simulink model "SimulinkSS"  (R2019a)
settings: Solver=FixedStepAuto  StartTime=0.0  StopTime=60  FixedStep=1e-2  RelTol=1e-3
undefined symbols (not defined in the file): G, K, Ki, x0_tf4
settings Model: Creator=luisg  LastModifiedBy=luisg

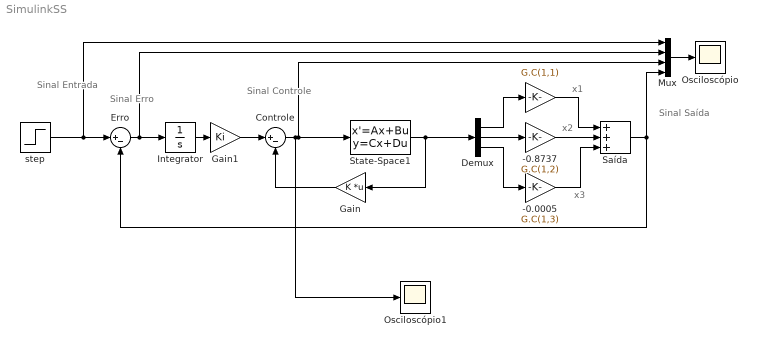
== system SimulinkSS ==
  note: Sinal
      | Entrada
  note: x1
  note: x2
  note: x3
  note: Sinal
      | Erro
  note: Sinal
      | Controle
  note: Sinal
      | Saída
  " " : Gain  Gain=G.C(1,1)
  -0.0005 : Gain  Gain=G.C(1,3)
  -0.8737 : Gain  Gain=G.C(1,2)
  Controle : Sum  Inputs=|+-
  Demux : Demux  Outputs=3
  Erro : Sum  Inputs=|+-
  Gain : Gain  Gain=K  Multiplication=Matrix(K*u)
  Gain1 : Gain  Gain=Ki
  Integrator : Integrator
  Mux : Mux
  Osciloscópio : Scope
  Osciloscópio1 : Scope
  Saída : Sum  Inputs=+++
  State-Space1 : StateSpace  A=G.A  B=G.B  C=[1 0 0; 0 1 0; 0 0 1]  D=[0;0;0]  InitialCondition=x0_tf4
  step : Step  Time=100  Before=70  After=70  SampleTime=0.05
  wires:
  Controle/1 -> State-Space1/1, Mux/3, Osciloscópio1/1
  Gain/1 -> Controle/2
  Erro/1 -> Mux/2, Integrator/1
  step/1 -> Mux/1, Erro/1
  State-Space1/1 -> Demux/1, Gain/1
  Demux/2 -> -0.8737/1
  Demux/3 -> -0.0005/1
  Demux/1 -> " "/1
  Saída/1 -> Mux/4, Erro/2
  Gain1/1 -> Controle/1
  Integrator/1 -> Gain1/1
  -0.8737/1 -> Saída/2
  " "/1 -> Saída/1
  -0.0005/1 -> Saída/3
  Mux/1 -> Osciloscópio/1
